simulink model "DHT22"  (R2019b)
settings: Solver=FixedStepAuto  StartTime=0.0  StopTime=inf  FixedStep=0.1  RelTol=1e-3  EnableMultiTasking=on
libraries: arduinolib x2, Arduino_Additional_Lib x1
settings Model: SimulationMode=external  ExtModeTrigDuration=2  Creator=TNiederhauser  LastModifiedBy=TNiederhauser
settings DataIOCC: ReturnWorkspaceOutputs=off
settings OptimizationCC: EnhancedBackFolding=on  PassReuseOutputArgsThreshold=0  MaxStackSize=64  OptimizeBlockOrder=speed  DifferentSizesBufferReuse=on  OptimizationCustomize=off
settings DebuggingCC: ParameterTunabilityLossMsg=error  ArithmeticOperatorsInVariantConditions=warning
settings HardwareCC: ProdBitPerInt=16  ProdBitPerPointer=16  ProdBitPerSizeT=16  ProdBitPerPtrDiffT=16  ProdLargestAtomicFloat=None  ProdWordSize=8  ProdHWDeviceType=Atmel->AVR  UseEmbeddedCoderFeatures=off
settings SFSimCC: SimUseLocalCustomCode=off  MATLABDynamicMemAlloc=off  CustomCodeUndefinedFunction=UseInterfaceOnly
settings RTWCC: SystemTargetFile=ert.tlc  HardwareBoard=Arduino Uno  TLCOptions=-aInlineSetEventsForThisBaseRateFcn=TLC_FALSE -aSuppressMultiTaskScheduler=TLC_FALSE -aRateBasedStepFcn=1  TemplateMakefile=ert_default_tmf  GenerateReport=on  RTWUseLocalCustomCode=off  Toolchain=Arduino AVR  BuildConfiguration=Faster Runs  LaunchReport=on
settings CodeAppCC: ForceParamTrailComments=on  OperatorAnnotations=on
settings ERTTargetCC: ERTCustomFileBanners=off  SupportContinuousTime=on  SupportNonInlinedSFcns=on  RemoveResetFunc=off  SupportVariableSizeSignals=on  ModelStepFunctionPrototypeControlCompliant=off  ExtModeStaticAllocSize=250

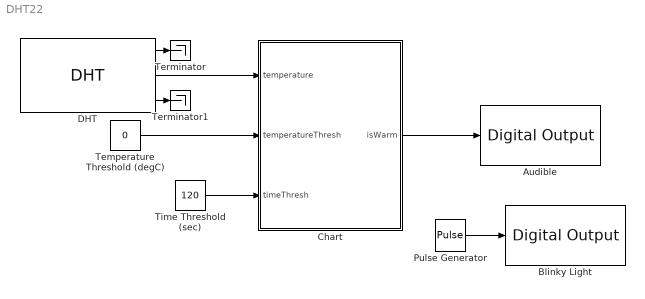
== system DHT22 ==
  Audible : arduinolib/Digital Output  pinNumber=4  blockPlatform=arduino
  Blinky Light : arduinolib/Digital Output  pinNumber=13  blockPlatform=arduino
  Chart : Stateflow chart  BlockKeywords=__PRM__SERIALIZED__DATA__:Stateflow Chart,Stateflow Diagram  TreatAsAtomicUnit=on
  DHT : Arduino_Additional_Lib/DHT  F=off  Pin=2  Tp=22  Ts=2
      settings: SourceProductName=Arduino Additional Sensors Library
  Pulse Generator : DiscretePulseGenerator  PulseType=Time based  PulseWidth=50
  Temperature Threshold (degC) : Constant  Value=0
  Terminator : Terminator
  Terminator1 : Terminator
  Time Threshold (sec) : Constant  Value=120
  wires:
  DHT/2 -> Chart/1(temperature)
  DHT/1 -> Terminator/1
  DHT/3 -> Terminator1/1
  Pulse Generator/1 -> Blinky Light/1
  Chart/1(isWarm) -> Audible/1
  Temperature Threshold (degC)/1 -> Chart/2(temperatureThresh)
  Time Threshold (sec)/1 -> Chart/3(timeThresh)

== stateflow chart DHT22/Chart ==
  state ColdAndHappy
    entry: isWarm = 0;
  state Undecided
  state TooWarm
    entry: isWarm = 1;
  (default) -> ColdAndHappy
  ColdAndHappy -> Undecided : [temperature > temperatureThresh]
  Undecided -> TooWarm [order 1] : after(timeThresh, sec)
  Undecided -> ColdAndHappy [order 2] : [temperature <= temperatureThresh]
  TooWarm -> ColdAndHappy : [temperature <= temperatureThresh]
  data: temperature input; temperatureThresh input; isWarm output; timeThresh input
